simulink library "Idq_controller_lib"  (R2014b)
settings: Solver=ode45  StartTime=0.0  StopTime=10.0  RelTol=1e-3
values from neighbouring files (symbols this model uses):
  f = 60    [global_parameters.m]
  L = Vdc_nom/(IacRMS*0.2/(2/fs))    [BES_init.m]
  Tds = Ts    (= 8e-05)    [global_parameters.m]
undefined symbols (not defined in the file): I_ki, I_kp, Id_at_max, Iq_at_max, Vdc_nom
settings Model: Creator=CH24070  LastModifiedBy=CH24070

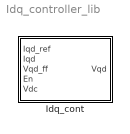
== system Idq_controller_lib ==
  Idq_cont : Subsystem  mask{L=L, iq_max=Iq_at_max, id_max=Id_at_max, kp=I_kp, ki=I_ki, Vdc_nom=Vdc_nom}
      mask prompts: L "Boost Inductor"; iq_max "Maximum Iq"; id_max "Maximum Id"; kp "Proportional Gain"; ki "Integral Gain"; Vdc_nom "Nominal DC Bus Voltage"
      mask init:
      | global_parameters

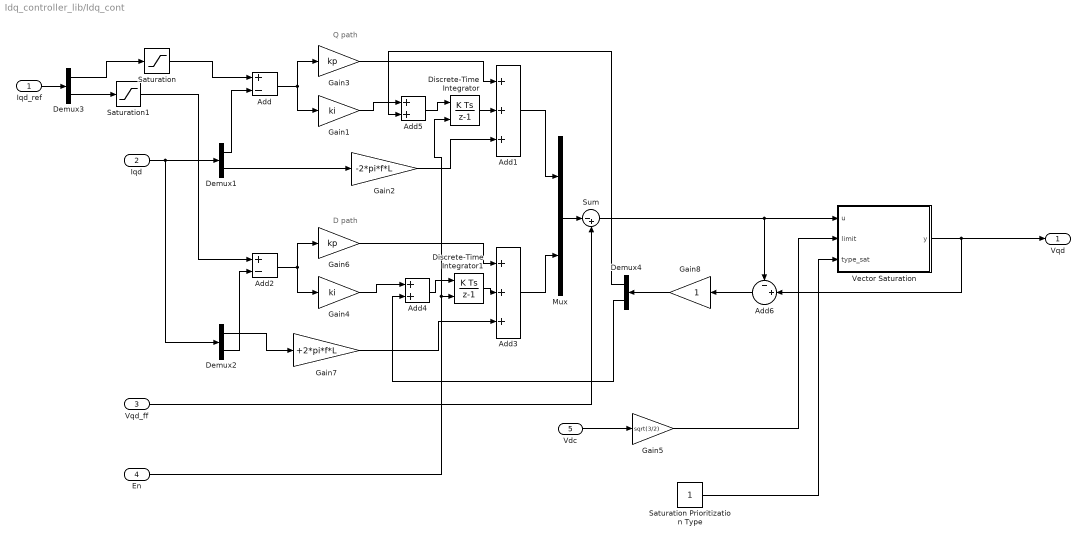
== system Idq_controller_lib/Idq_cont ==
  note: Q path
  note: D path
  Iqd_ref : Inport
  Iqd : Inport  Port=2
  Vqd_ff : Inport  Port=3  PortDimensions=2
  En : Inport  Port=4  OutDataTypeStr=boolean  PortDimensions=1
  Vdc : Inport  Port=5  PortDimensions=1
  Add : Sum  Inputs=+-
  Add1 : Sum  Inputs=+++
  Add2 : Sum  Inputs=+-
  Add3 : Sum  Inputs=+++
  Add4 : Sum
  Add5 : Sum
  Add6 : Sum  Inputs=-+|
  Demux{1..4} (4 alike) : Demux  Outputs=2
  Discrete-Time Integrator : DiscreteIntegrator  ExternalReset=rising  InitialConditionSetting=State (most efficient)  SampleTime=Tds
  Discrete-Time Integrator1 : DiscreteIntegrator  ExternalReset=rising  InitialConditionSetting=State (most efficient)  SampleTime=Tds
  Gain1 : Gain  Gain=ki
  Gain2 : Gain  Gain=-2*pi*f*L
  Gain3 : Gain  Gain=kp
  Gain4 : Gain  Gain=ki
  Gain5 : Gain  Gain=sqrt(3/2)
  Gain6 : Gain  Gain=kp
  Gain7 : Gain  Gain=+2*pi*f*L
  Gain8 : Gain
  Mux : Mux  Inputs=2
  Saturation : Saturate  UpperLimit=iq_max  LowerLimit=-iq_max
  Saturation Prioritization Type : Constant
  Saturation1 : Saturate  UpperLimit=id_max  LowerLimit=-id_max
  Sum : Sum  Inputs=|-+
  Vector Saturation : MATLAB Function  TreatAsAtomicUnit=on
  Vqd : Outport
  wires:
  Add/1 -> Gain1/1, Gain3/1
  Gain6/1 -> Add3/1
  Demux4/2 -> Add4/2
  Mux/1 -> Sum/1
  Discrete-Time Integrator1/1 -> Add3/2
  Gain7/1 -> Add3/3
  Demux2/2 -> Add2/2
  Add3/1 -> Mux/2
  En/1 -> Discrete-Time Integrator1/2, Discrete-Time Integrator/2
  Gain1/1 -> Add5/1
  Gain2/1 -> Add1/3
  Demux3/2 -> Saturation1/1
  Discrete-Time Integrator/1 -> Add1/2
  Iqd/1 -> Demux2/1, Demux1/1
  Add4/1 -> Discrete-Time Integrator1/1
  Demux3/1 -> Saturation/1
  Add5/1 -> Discrete-Time Integrator/1
  Gain4/1 -> Add4/1
  Add1/1 -> Mux/1
  Sum/1 -> Vector Saturation/1(u), Add6/1
  Gain3/1 -> Add1/1
  Demux1/1 -> Add/2
  Vector Saturation/1(y) -> Vqd/1, Add6/2
  Demux1/2 -> Gain2/1
  Add2/1 -> Gain4/1, Gain6/1
  Gain8/1 -> Demux4/1
  Iqd_ref/1 -> Demux3/1
  Saturation1/1 -> Add2/1
  Saturation/1 -> Add/1
  Demux4/1 -> Add5/2
  Demux2/1 -> Gain7/1
  Vqd_ff/1 -> Sum/2
  Saturation Prioritization Type/1 -> Vector Saturation/3(type_sat)
  Gain5/1 -> Vector Saturation/2(limit)
  Add6/1 -> Gain8/1
  Vdc/1 -> Gain5/1

== matlab function Idq_controller_lib/Idq_cont/Vector Saturation ==
  data: u input; y output; limit input; type_sat input
function y = fcn(u, limit, type_sat)
% When the magnitude is of u is greater than limit prioritize the
% saturation to u(type_sat) dimension.  u is two dimensional input.
%#codegen
y=zeros(2,1); % required initialization
u_sign=sign(u);

if(abs(u(1)) > limit)
    u(1) = u_sign(1).*limit;
end
if(abs(u(2)) > limit)
    u(2) =  u_sign(2).*limit;
end
if(u(1)^2 + u(2)^2 > limit^2)
    if(type_sat == 1) % priority given to u(1)
        y(1) = u(1);
        y(2) = u_sign(2) .* sqrt(limit^2 - u(1)^2); 
    else  % priority given to u(2)
        y(2) = u(2);
        y(1) =  u_sign(1) .* sqrt(limit^2 - u(2)^2); 
    end
else
    y = u;
end
